simulink model "ADAS_Main_ClosedLoop"  (R2026a)
settings: Solver=FixedStepDiscrete  StopTime=20
InitFcn:
  | createLidarActorProfiles;
  | % L3/L4 closed-loop ego initial condition, READ FROM THE TEST-1 FIXTURE
  | % (not hard-coded in the vehicle model, which stays reusable)
  | clS = load('D:\AutonomousDriving\D_scenarios\V2_0_ClosedLoop_Test9_TwoObstacles_WideRoad.mat');
  | clA = clS.data.ActorSpecifications([clS.data.ActorSpecifications.ActorID] == clS.data.EgoCarId);
  | CL_EGO_IC = [clA.Position(1); clA.Position(2); clA.Yaw*pi/180; clA.Speed(1)];
  | clear clS clA
  | % Non-virtual ego-pose bus type. A MATLAB Function block (Extract_Ego_Kinematics)
  | % cannot accept a VIRTUAL bus, so the Bus Creator must emit a defined Simulink.Bus.
  | % Shape copied from the installed validator contract and from BusActorsActors.
  | clN = {'ActorID','Position','Velocity','Roll','Pitch','Yaw','AngularVelocity'};
  | clD = {[1 1],[1 3],[1 3],[1 1],[1 1],[1 1],[1 3]};
  | clEls = Simulink.BusElement.empty(0,1);
  | for clI = 1:7
  |   clE = Simulink.BusElement; clE.Name = clN{clI}; clE.Dimensions = clD{clI}; clE.DataType = 'double';
  |   clEls(clI,1) = clE;
  | end
  | BusEgoPose_CL = Simulink.Bus; BusEgoPose_CL.Elements = clEls;
  | clear clN clD clEls clE clI
StopFcn:
  | cl_plot_closedloop_trajectory;
model workspace (MAT data in the model file):
  firstWarning = 1
  originalScenarioChecksum = '71EAF3DF157DF5A35F75811B676F8B0F'
undefined symbols (not defined in the file): driving, matlabshared
libraries: drivingscenarioandsensors x3, lidarlib x1
(part 4 of 7)

== matlab function ADAS_Main_ClosedLoop/Tracking_Prediction/Track_Update ==
  data: pState input; oState output; pCov input; pID input; pStatus input; pNextID input; prevHits input uint32 size=512 1; prevTsu input double size=512 1; prevR1 input double size=512 3; trkAssign input; fusedObjects input; numFusedObjects input; oCov output; oID output; oStatus output; oNextID output; oHits output; oTsu output; oR1 output; updDiag output; egoTransform input; prevAttr input double size=512 3; oAttr output
function [oState, oCov, oID, oStatus, oNextID, oHits, oTsu, oR1, updDiag, oAttr] = ...
    Track_Update(pState, pCov, pID, pStatus, pNextID, prevHits, prevTsu, prevR1, ...
                 trkAssign, fusedObjects, numFusedObjects, egoTransform, prevAttr)
%#codegen
% TRACK_UPDATE  Stage 4: matched measurement update + new-track initialization.
%   This is the stage that CLOSES the state feedback loop for the first time.
%
% THIS BLOCK DOES NOT: confirm, coast, delete, transfer to a lost table, apply
% T_lost, keep history, estimate acceleration, emit prediction horizons, or make
% any lifecycle decision. Those are Stage 5+.
%
% VELOCITY OBSERVATION IS DELIBERATELY NOT IMPLEMENTED - see the block report.
% FusedObjects cols 9..13 carry velocity, but integrating it as a measurement
% needs design decisions that are NOT frozen at implementation level (joint vs
% sequential update, the absent position/velocity cross-covariance, and what a
% Radar velocity on hit 1 or hit 2 should do to the frozen initialisation and
% two-point constructions). Choosing silently is forbidden, so Stage 4
% implements only the MANDATORY position update + two-point velocity init.
%
% ORDER (frozen): previous state -> ego compensation -> CV prediction ->
%   association -> matched update / two-point -> new-track init -> Unit Delay.
% New tracks are created AFTER matching, so they are never associated in the
% same frame they are born.
%
% MEASUREMENT UPDATE (3rd and later hits)
%   H = [1 0 0 0; 0 1 0 0]
%   S = H*Ppred*H' + R          <-- R ONLY. The association wander term
%                                   W = 0.40^2*I is NEVER used here, and the
%                                   LiDAR D^2/12 term is NOT re-applied; it is
%                                   already inside the fused R where applicable.
%   K = Ppred*H'*inv(S)         analytic 2x2 inverse, isPD2 guarded
%   xPost = xPred + K*(z - H*xPred)
%   JOSEPH FORM: A = I - K*H ;  PPost = A*Ppred*A' + K*R*K'
%   then symmetrise -> floor -> PD check -> reset if required.
%   Covariance is never scalarised; XY/XV/YV correlations are preserved.
%
% FIRST-HIT INITIALISATION (frozen)
%   x = [z.x; z.y; 0; 0]   -- the velocity zeros are PLACEHOLDERS, NOT a
%                             measurement and NOT "stationary".
%   P = [ R      0        ;  0   SIGMA_V0^2*I ] ,  SIGMA_V0 = 40 m/s
%   Pxv = 0 ;  VelocityConverged = false.
%   FusedObjects velocity is NEVER read here, so a VelUnobserved zero can never
%   be mistaken for a stationary measurement.
%
% CORRECTION 1 - R1 FRAME CONSISTENCY
%   R1 is stored when the track is born, in THAT frame. The stored value is now
%   rotated every frame by the SAME T the ego compensation applies to the state,
%   so R1 always lives in the CURRENT ego frame and composes correctly across a
%   multi-frame gap. No accumulated-rotation state is needed.
%       R1 <- T * R1 * T'   each frame,  T = [c s; -s c], c=cos(dpsi), s=sin(dpsi)
%   Rotation is orthogonal, so this is exact: it preserves R1's eigenvalues and
%   only re-expresses them in the current frame. For isotropic R1 it is a no-op.
%
% CORRECTION 2 - INVALID COVARIANCE NEVER INITIALISES A TRACK
%   A detection whose position covariance is non-PD, NaN or Inf is REJECTED for
%   new-track initialization and counted in nInitRejected. No covariance is
%   invented and an invalid measurement is never treated as near-zero
%   uncertainty. (Matched-track handling is unchanged: the update is skipped,
%   the predicted state is kept, and nUpdateRejected counts it.)
%
% CORRECTION 3 - POSITION FLOOR AT VALID INITIALIZATION
%   Rz -> symmetrise -> floor at P_FLOOR_POS -> PD validation -> store.
%   A legitimately tiny covariance (e.g. 1e-12) can no longer bypass the frozen
%   positional floor. Valid covariance is never replaced, only floored.
%
% SECOND-HIT TWO-POINT CONSTRUCTION (frozen) - REPLACES the Kalman update
%   position = z2
%   velocity = (z2 - z1)/dt_elapsed
%   Ppos = R2 ;  Pxv = R2/dt_elapsed ;  Pvv = (R1 + R2)/dt_elapsed^2
%   Exact form, NOT 2*R/dt^2. Uses the real elapsed time, not a hard-coded 0.1.
%
% NEW FIXED-SIZE STATE ADDED BY STAGE 4 (the minimum the two-point needs)
%   oHits [512x1] uint32  measurement-update count per slot
%   oTsu  [512x1] double  seconds since that slot's last update
%   oR1   [512x3] double  first-observation covariance [Rxx Ryy Rxy], rotated
%                         into the current ego frame every step (correction 1)
%
% STAGE-4 TEMPORARY STATUS CODES - NOT the frozen lifecycle codes
%   0 = free slot
%   1 = active (pre-lifecycle). Stage 5 will redefine this field entirely;
%       nothing here should be read as tentative/confirmed/coasted/lost.
%
% UNMATCHED ACTIVE TRACKS keep their Stage-2 predicted state untouched and are
% only counted. No coasting, no deletion, no fake measurement.
%
% OVERFLOW: if no free slot exists, NO existing track is evicted. The detection
% is simply not admitted, TrackTableOverflow is raised and NumTracksDropped
% increments.
%
% Diagnostics are diagnostics: a LowMargin or DisplacedAssignment assignment is
% still updated normally. They never reject an update.
%
% SCENARIO INDEPENDENCE: consumes only predicted track state, the association
% result and fused detections. No actor identity, class, count, trajectory, map
% or scenario geometry.

MAX_T = 512;
MAX_D = 356;
DT    = 0.1;

P_FLOOR_POS = 1e-6;
P_FLOOR_VEL = 1e-7;
SIGMA_V0    = 40.0;
V_CONV      = 0.875;

C_VALID = 1; C_X = 2; C_Y = 3; C_CXX = 5; C_CYY = 6; C_CXY = 7;

% ---- Stage 8: Radar scalar radial-velocity observation -------------------
C_VX = 9; C_VY = 10; C_VXX = 11; C_VYY = 12; C_VXY = 13; C_FLAGS = 27;

% ---- persistent LiDAR extent attributes (additive; no algorithm change) ----
% Carried VERBATIM from FusedObjects. Tracking does not interpret them: the
% bits keep their LiDAR ObservationFlags meanings (1 Sparse, 2 DegenerateShape,
% 4 ThinFootprint, 8 ExtentUntrusted). No extent is ever invented here, and no
% default size is ever substituted - a slot with no observation keeps zeros.
C_LEN = 14; C_WID = 15; C_LFLAGS = 26;
FLAG_VEL_RADAR = uint32(32);        % FusionFlags bit 32 = VelFromRadar
%
% RATIO_MIN is a SEMANTIC COVARIANCE-SHAPE GUARD, not a Radar-quality
% threshold. Its only job is to detect a reported velocity covariance that is
% NOT of the expected "one observed direction + placeholder" shape, in which
% case the premise that Radar observes exactly one scalar along the minor
% eigenvector does not describe that report and must not be imposed on it.
% It is NOT a numerical-conditioning guard: the closed-form extraction below
% was measured accurate to 1.2e-6 deg at every ratio down to 1.0001, with
% Rayleigh-quotient excess <= 1.9e-8 there and <= 1e-16 for ratio >= 2.
% 4 = a 2x separation in sigma, the weakest statement that still means
% "meaningfully anisotropic". With the verified lambda_max = crossVelSig^2 =
% 100 this corresponds to sigma_rr <= 5 m/s and rejects 0 of 65 Radar rows in
% the reference scenario; it is NOT tuned to that scenario, and the earlier
% 1%-Fisher-information argument for 100 was WITHDRAWN as invalid, because the
% discarded channel is a hard-coded placeholder whose information is fictitious.
RATIO_MIN = 4.0;
%
% Mirrors Tracking_State_Update's own YAW_EPS = 1e-6 rad/s branch. That block
% tests |yawRate| <= YAW_EPS; here only dpsi = yawRate*DT is available, so the
% equivalent test is |dpsi| <= YAW_EPS*DT. Same branch, same numbers.
YAW_EPS_DT = 1e-6 * 0.1;
%
% Velocity gate, 1 degree of freedom - the dimension of the INNOVATION, not of
% the state and not of the velocity vector. chi2(1,0.99) = 6.635, set to the
% same 0.99 confidence level as the frozen position gate. ENGINEERING CHOICE;
% NOT empirically calibrated from this scenario (0 consistency failures in 1917
% rows gives no outlier rate to calibrate against).
CHI2_V1   = 6.635;

oState  = zeros(MAX_T,4);
oCov    = zeros(MAX_T,10);
oID     = zeros(MAX_T,1,'uint32');
oStatus = zeros(MAX_T,1,'uint8');
oHits   = zeros(MAX_T,1,'uint32');
oTsu    = zeros(MAX_T,1);
oR1     = zeros(MAX_T,3);
oAttr   = zeros(MAX_T,3);        % [Length Width LiDARFlags] per SLOT
oNextID = pNextID;
if oNextID < 1
    oNextID = uint32(1);
end
updDiag = zeros(1,26);   % 1..13 unchanged from Stage 4; 14..26 are Stage 8

nD = double(numFusedObjects);
if nD < 0,     nD = 0;     end
if nD > MAX_D, nD = MAX_D; end

% ---- ego rotation for this step (same T the state compensation used) -----
dpsiE = egoTransform(3);
if ~isfinite(dpsiE), dpsiE = 0; end
cE =  cos(dpsiE);  sE = sin(dpsiE);
t11 =  cE; t12 = sE;
t21 = -sE; t22 = cE;

% ---- Stage 8: EXACT ego speed recovered from egoTransform -----------------
% No new input and no new port: egoTransform already carries (dx, dy, dpsi).
% Tracking_State_Update forms the displacement on the frozen constant-turn-rate
% arc, so with chord c = |[dx;dy]| = 2*(v/w)*|sin(dpsi/2)| and arc length v*dt,
%     v = (c/dt) * (dpsi/2) / sin(dpsi/2)
% exactly. The factor is even in dpsi and tends to 1, so the sign of dpsi is
% irrelevant. The branch below MIRRORS the producer's own branch: when
% |yawRate| <= YAW_EPS it writes dx = v*dt, dy = 0, and |dpsi| = |yawRate|*dt,
% so the equivalent test here is |dpsi| <= YAW_EPS*DT and then v = c/dt EXACTLY.
% Verified against egoKin over the scenario: max error 3.553e-15 m/s. The
% chord-only shortcut c/dt would err by 7.978e-04 m/s, so it is NOT used.
dxE = egoTransform(1);
dyE = egoTransform(2);
if ~isfinite(dxE), dxE = 0; end
if ~isfinite(dyE), dyE = 0; end
cEgo = sqrt(dxE*dxE + dyE*dyE);
if abs(dpsiE) > YAW_EPS_DT
    egoSpeed = (cEgo/DT) * (dpsiE/2) / sin(dpsiE/2);
else
    egoSpeed = cEgo/DT;
end
if ~isfinite(egoSpeed) || egoSpeed < 0, egoSpeed = 0; end

% ---- carry the predicted state forward as the default --------------------
nActIn = 0;
for t = 1:MAX_T
    oStatus(t) = pStatus(t);
    oID(t)     = pID(t);
    oHits(t)   = prevHits(t);
    a11 = prevR1(t,1); a22 = prevR1(t,2); a12 = prevR1(t,3);
    m11 = t11*a11 + t12*a12;  m12 = t11*a12 + t12*a22;
    m21 = t21*a11 + t22*a12;  m22 = t21*a12 + t22*a22;
    oR1(t,1) = m11*t11 + m12*t12;
    oR1(t,3) = m11*t21 + m12*t22;
    oR1(t,2) = m21*t21 + m22*t22;
    if pStatus(t) == 0
        oTsu(t) = 0;
        continue
    end
    nActIn = nActIn + 1;
    oTsu(t) = prevTsu(t) + DT;          % prediction for this frame already ran
    for c = 1:3
        oAttr(t,c) = prevAttr(t,c);     % persist; a coasted track keeps its last extent
    end
    for k = 1:4
        oState(t,k) = pState(t,k);
    end
    for k = 1:10
        oCov(t,k) = pCov(t,k);
    end
end

detUsed = false(MAX_D,1);
nMatch = 0; nTwoPt = 0; nFloor = 0; nReset = 0; nRej = 0;

% ---- Stage 8 velocity-observation counters ------------------------------
nVCand = 0; nVObs = 0; nVGate = 0; nVCov = 0; nVDeg = 0; nVPD = 0;
rMin = 0; rMax = 0; rB = zeros(1,6);

% ---- matched update ------------------------------------------------------
% NOTE on the two-point construction: z1 is NOT stored separately. After the
% first hit the state is [z1x z1y 0 0]; with zero velocity the CV prediction
% does not move it, so the predicted position pState(t,1:2) IS z1 already
% ego-compensated into the CURRENT frame. Using it is more correct than storing
% a raw z1 that would be expressed in a stale frame.
% R1 is stored in the frame it was measured; the frozen formula does not
% prescribe rotating it, and over one step the ego rotation is <= 0.036 rad in
% this scenario, so it is applied literally as frozen. Documented, not silently
% changed.
for t = 1:MAX_T
    if pStatus(t) == 0, continue; end
    if trkAssign(t,1) ~= 1, continue; end
    j = trkAssign(t,3);
    if j < 1 || j > nD, continue; end
    if fusedObjects(j,C_VALID) ~= 1, continue; end

    r11 = fusedObjects(j,C_CXX); r22 = fusedObjects(j,C_CYY); r12 = fusedObjects(j,C_CXY);
    if ~isPD2(r11, r22, r12)
        nRej = nRej + 1;
        continue
    end
    zx = fusedObjects(j,C_X); zy = fusedObjects(j,C_Y);
    detUsed(j) = true;
    nMatch = nMatch + 1;

    P = zeros(4,4);
    P(1,1)=pCov(t,1); P(1,2)=pCov(t,2); P(1,3)=pCov(t,3); P(1,4)=pCov(t,4);
    P(2,2)=pCov(t,5); P(2,3)=pCov(t,6); P(2,4)=pCov(t,7);
    P(3,3)=pCov(t,8); P(3,4)=pCov(t,9); P(4,4)=pCov(t,10);
    P(2,1)=P(1,2); P(3,1)=P(1,3); P(4,1)=P(1,4);
    P(3,2)=P(2,3); P(4,2)=P(2,4); P(4,3)=P(3,4);

    x1 = pState(t,1); x2 = pState(t,2); x3 = pState(t,3); x4 = pState(t,4);
    okUpd = true;

    if prevHits(t) == 1
        dte = oTsu(t);
        if ~(dte > 0), dte = DT; end
        q11 = oR1(t,1); q22 = oR1(t,2); q12 = oR1(t,3);   % frame-consistent
        vX = (zx - x1)/dte;
        vY = (zy - x2)/dte;
        P = zeros(4,4);
        P(1,1) = r11;      P(1,2) = r12;      P(2,1) = r12;      P(2,2) = r22;
        P(1,3) = r11/dte;  P(3,1) = P(1,3);
        P(1,4) = r12/dte;  P(4,1) = P(1,4);
        P(2,3) = r12/dte;  P(3,2) = P(2,3);
        P(2,4) = r22/dte;  P(4,2) = P(2,4);
        P(3,3) = (q11 + r11)/(dte*dte);
        P(4,4) = (q22 + r22)/(dte*dte);
        P(3,4) = (q12 + r12)/(dte*dte);  P(4,3) = P(3,4);
        x1 = zx; x2 = zy; x3 = vX; x4 = vY;
        nTwoPt = nTwoPt + 1;
    else
        s11 = P(1,1) + r11; s22 = P(2,2) + r22; s12 = P(1,2) + r12;
        if ~isPD2(s11, s22, s12)
            nRej = nRej + 1; okUpd = false;
        else
            dS = s11*s22 - s12*s12;
            i11 =  s22/dS; i22 =  s11/dS; i12 = -s12/dS;
            K = zeros(4,2);
            for a = 1:4
                K(a,1) = P(a,1)*i11 + P(a,2)*i12;
                K(a,2) = P(a,1)*i12 + P(a,2)*i22;
            end
            y1 = zx - x1; y2 = zy - x2;
            x1 = x1 + K(1,1)*y1 + K(1,2)*y2;
            x2 = x2 + K(2,1)*y1 + K(2,2)*y2;
            x3 = x3 + K(3,1)*y1 + K(3,2)*y2;
            x4 = x4 + K(4,1)*y1 + K(4,2)*y2;
            A = eye(4);
            for a = 1:4
                A(a,1) = A(a,1) - K(a,1);
                A(a,2) = A(a,2) - K(a,2);
            end
            Rm = [r11 r12; r12 r22];
            P = A*P*A' + K*Rm*K';
        end
    end

    if ~okUpd
        detUsed(j) = false; nMatch = nMatch - 1;
        continue
    end

    % ---- STAGE 8: Radar scalar radial-velocity update --------------------
    % MANDATORY ORDER. Position update (else-branch) or two-point
    % RECONSTRUCTION (prevHits==1 branch) has already completed above; the
    % radial update runs strictly after it and never replaces it. The
    % two-point step deliberately builds the Pxv structure this update then
    % exploits: K's upper block is Pxv/S, so a velocity observation also
    % corrects POSITION whenever Pxv ~= 0. Reversing the order would destroy
    % the reconstruction, so the order is load-bearing and is NOT licensed by
    % the position/velocity order-equivalence that holds for two genuine
    % measurement updates.
    if bitand(uint32(fusedObjects(j,C_FLAGS)), FLAG_VEL_RADAR) > 0
        nVCand = nVCand + 1;
        [x1, x2, x3, x4, Pv, cdV, ratV] = radialVelUpd( ...
            x1, x2, x3, x4, P, ...
            fusedObjects(j,C_VX),  fusedObjects(j,C_VY), ...
            fusedObjects(j,C_VXX), fusedObjects(j,C_VYY), fusedObjects(j,C_VXY), ...
            RATIO_MIN, CHI2_V1, egoSpeed);
        if ratV > 0
            if rMax == 0
                rMin = ratV; rMax = ratV;
            else
                if ratV < rMin, rMin = ratV; end
                if ratV > rMax, rMax = ratV; end
            end
            bi = ratioBucket(ratV);
            rB(bi) = rB(bi) + 1;
        end
        if cdV == 0
            P = Pv;  nVObs = nVObs + 1;
        elseif cdV == 2
            nVDeg = nVDeg + 1;          % shape guard: not the expected shape
        elseif cdV == 3
            nVGate = nVGate + 1;        % rejects ONLY the velocity update
        else
            nVCov = nVCov + 1;          % invalid / non-finite covariance
        end
    end

    P = (P + P')/2;
    fl = 0; rs = 0;
    if P(1,1) < P_FLOOR_POS, P(1,1) = P_FLOOR_POS; fl = 1; end
    if P(2,2) < P_FLOOR_POS, P(2,2) = P_FLOOR_POS; fl = 1; end
    if P(3,3) < P_FLOOR_VEL, P(3,3) = P_FLOOR_VEL; fl = 1; end
    if P(4,4) < P_FLOOR_VEL, P(4,4) = P_FLOOR_VEL; fl = 1; end
    if ~(isPD2(P(1,1),P(2,2),P(1,2)) && isPD2(P(3,3),P(4,4),P(3,4)))
        d1=P(1,1); d2=P(2,2); d3=P(3,3); d4=P(4,4);
        if ~isfinite(d1) || d1 < P_FLOOR_POS, d1 = P_FLOOR_POS; end
        if ~isfinite(d2) || d2 < P_FLOOR_POS, d2 = P_FLOOR_POS; end
        if ~isfinite(d3) || d3 < P_FLOOR_VEL, d3 = P_FLOOR_VEL; end
        if ~isfinite(d4) || d4 < P_FLOOR_VEL, d4 = P_FLOOR_VEL; end
        P = zeros(4,4); P(1,1)=d1; P(2,2)=d2; P(3,3)=d3; P(4,4)=d4;
        rs = 1;
    end
    nFloor = nFloor + fl; nReset = nReset + rs;

    oState(t,1)=x1; oState(t,2)=x2; oState(t,3)=x3; oState(t,4)=x4;
    oCov(t,1)=P(1,1); oCov(t,2)=P(1,2); oCov(t,3)=P(1,3); oCov(t,4)=P(1,4);
    oCov(t,5)=P(2,2); oCov(t,6)=P(2,3); oCov(t,7)=P(2,4);
    oCov(t,8)=P(3,3); oCov(t,9)=P(3,4); oCov(t,10)=P(4,4);
    oHits(t) = prevHits(t) + uint32(1);
    oTsu(t)  = 0;
    oAttr(t,1) = fusedObjects(j,C_LEN);      % matched path: refresh verbatim
    oAttr(t,2) = fusedObjects(j,C_WID);
    oAttr(t,3) = fusedObjects(j,C_LFLAGS);
end

% ---- new-track initialization from unmatched valid detections ------------
% No threat, distance or semantic ranking. No dropping on SupportScore.
% Deterministic lowest-free-slot allocation. Never evicts an existing track.
nNew = 0; nDrop = 0; ovf = 0; nInitRej = 0;
for j = 1:nD
    if detUsed(j), continue; end
    if fusedObjects(j,C_VALID) ~= 1, continue; end
    r11 = fusedObjects(j,C_CXX); r22 = fusedObjects(j,C_CYY); r12 = fusedObjects(j,C_CXY);
    if ~isPD2(r11, r22, r12)
        nInitRej = nInitRej + 1;        % REJECT - never invent a covariance
        continue
    end
    if r11 < P_FLOOR_POS, r11 = P_FLOOR_POS; end   % floor, then re-validate
    if r22 < P_FLOOR_POS, r22 = P_FLOOR_POS; end
    if ~isPD2(r11, r22, r12)
        nInitRej = nInitRej + 1;
        continue
    end
    slot = 0;
    for t = 1:MAX_T
        if oStatus(t) == 0, slot = t; break; end
    end
    if slot == 0
        ovf = 1; nDrop = nDrop + 1;                      % NO EVICTION
        continue
    end
    oState(slot,1) = fusedObjects(j,C_X);
    oState(slot,2) = fusedObjects(j,C_Y);
    oState(slot,3) = 0;                                  % PLACEHOLDER, not a
    oState(slot,4) = 0;                                  % measurement
    oCov(slot,1)  = r11; oCov(slot,2) = r12; oCov(slot,3) = 0; oCov(slot,4) = 0;
    oCov(slot,5)  = r22; oCov(slot,6) = 0;   oCov(slot,7) = 0;
    oCov(slot,8)  = SIGMA_V0*SIGMA_V0;
    oCov(slot,9)  = 0;
    oCov(slot,10) = SIGMA_V0*SIGMA_V0;
    oStatus(slot) = uint8(1);
    oID(slot)     = oNextID;
    oNextID       = oNextID + uint32(1);
    oHits(slot)   = uint32(1);
    oTsu(slot)    = 0;
    oR1(slot,1)   = r11; oR1(slot,2) = r22; oR1(slot,3) = r12;
    oAttr(slot,1) = fusedObjects(j,C_LEN);   % newborn path: attributes immediately
    oAttr(slot,2) = fusedObjects(j,C_WID);
    oAttr(slot,3) = fusedObjects(j,C_LFLAGS);

    % ---- STAGE 8: the NORMAL scalar update acting on the frozen prior ----
    % Every initialization line above is UNCHANGED. This is not a second
    % initialization path and not special-case init code: it is the same
    % radialVelUpd used by the matched loop, applied to the uninformative
    % prior that initialization just declared. Vx=Vy=0 with Pvv=40^2*I remains
    % the literal frozen init; the observation then reduces uncertainty along
    % the LOS only. Because Pxv = 0 at initialization, K(1) = K(2) = 0
    % EXACTLY, so the initialized position cannot be moved by this update.
    % On hit 1 the prior is uninformative (S ~ 1600 + sigma_r^2), so the gate
    % cannot reject: correct behaviour from an uninformative prior, not a bug.
    if bitand(uint32(fusedObjects(j,C_FLAGS)), FLAG_VEL_RADAR) > 0
        nVCand = nVCand + 1;
        Pi = zeros(4,4);
        Pi(1,1) = oCov(slot,1);  Pi(1,2) = oCov(slot,2);  Pi(2,1) = Pi(1,2);
        Pi(2,2) = oCov(slot,5);
        Pi(3,3) = oCov(slot,8);  Pi(3,4) = oCov(slot,9);  Pi(4,3) = Pi(3,4);
        Pi(4,4) = oCov(slot,10);
        [b1, b2, b3, b4, Pn, cdV, ratV] = radialVelUpd( ...
            oState(slot,1), oState(slot,2), oState(slot,3), oState(slot,4), Pi, ...
            fusedObjects(j,C_VX),  fusedObjects(j,C_VY), ...
            fusedObjects(j,C_VXX), fusedObjects(j,C_VYY), fusedObjects(j,C_VXY), ...
            RATIO_MIN, CHI2_V1, egoSpeed);
        if ratV > 0
            if rMax == 0
                rMin = ratV; rMax = ratV;
            else
                if ratV < rMin, rMin = ratV; end
                if ratV > rMax, rMax = ratV; end
            end
            bi = ratioBucket(ratV);
            rB(bi) = rB(bi) + 1;
        end
        if cdV == 0
            Pn = (Pn + Pn')/2;
            if Pn(1,1) < P_FLOOR_POS, Pn(1,1) = P_FLOOR_POS; end
            if Pn(2,2) < P_FLOOR_POS, Pn(2,2) = P_FLOOR_POS; end
            if Pn(3,3) < P_FLOOR_VEL, Pn(3,3) = P_FLOOR_VEL; end
            if Pn(4,4) < P_FLOOR_VEL, Pn(4,4) = P_FLOOR_VEL; end
            if isPD2(Pn(1,1),Pn(2,2),Pn(1,2)) && isPD2(Pn(3,3),Pn(4,4),Pn(3,4))
                oState(slot,1) = b1; oState(slot,2) = b2;
                oState(slot,3) = b3; oState(slot,4) = b4;
                oCov(slot,1)=Pn(1,1); oCov(slot,2)=Pn(1,2); oCov(slot,3)=Pn(1,3);
                oCov(slot,4)=Pn(1,4); oCov(slot,5)=Pn(2,2); oCov(slot,6)=Pn(2,3);
                oCov(slot,7)=Pn(2,4); oCov(slot,8)=Pn(3,3); oCov(slot,9)=Pn(3,4);
                oCov(slot,10)=Pn(4,4);
                nVObs = nVObs + 1;
            else
                nVPD = nVPD + 1;        % DISCARD - keep the frozen init intact
            end
        elseif cdV == 2
            nVDeg = nVDeg + 1;
        elseif cdV == 3
            nVGate = nVGate + 1;
        else
            nVCov = nVCov + 1;
        end
    end

    nNew = nNew + 1;
end

% ---- diagnostics ---------------------------------------------------------
nActOut = 0; nConv = 0;
for t = 1:MAX_T
    if oStatus(t) == 0, continue; end
    nActOut = nActOut + 1;
    if sqrt(oCov(t,8)) < V_CONV && sqrt(oCov(t,10)) < V_CONV
        nConv = nConv + 1;                 % derived every frame, never latched
    end
end
updDiag(1)  = nActIn;
updDiag(2)  = nMatch;
updDiag(3)  = nActIn - nMatch;
updDiag(4)  = nNew;
updDiag(5)  = nActOut;
updDiag(6)  = nTwoPt;
updDiag(7)  = nFloor;
updDiag(8)  = nReset;
updDiag(9)  = nConv;
updDiag(10) = nDrop;
updDiag(11) = ovf;
updDiag(12) = nRej;
updDiag(13) = nInitRej;
% ---- Stage 8 velocity-observation diagnostics ---------------------------
updDiag(14) = nVCand;    % detections carrying VelFromRadar that reached the update
updDiag(15) = nVObs;     % radial updates actually applied
updDiag(16) = nVGate;    % rejected by the chi2(1,0.99) velocity gate
updDiag(17) = nVCov;     % invalid / non-finite reported velocity covariance
updDiag(18) = nVDeg;     % rejected by the semantic shape guard (ratio < RATIO_MIN)
updDiag(19) = nVPD;      % post-update PD validation failed at initialization
updDiag(20) = rMin;      % min observed lambda_max/lambda_min (0 if none)
updDiag(21) = rMax;      % max observed
updDiag(22) = rB(1);     % ratio <  1e1
updDiag(23) = rB(2);     % ratio in [1e1,1e2)
updDiag(24) = rB(3);     % ratio in [1e2,1e3)
updDiag(25) = rB(4);     % ratio in [1e3,1e4)
updDiag(26) = rB(5) + rB(6);   % ratio >= 1e4

end

% ===========================================================================
function b = ratioBucket(r)
% Fixed-size log10 histogram bucket for the eigenvalue-ratio diagnostic.
b = 1;
if     r >= 1e5, b = 6;
elseif r >= 1e4, b = 5;
elseif r >= 1e3, b = 4;
elseif r >= 1e2, b = 3;
elseif r >= 1e1, b = 2;
end
end

% ===========================================================================
function tf = isPD2(a, b, c)
% 2x2 symmetric [a c; c b] is positive definite iff a > 0 and det > 0.
tf = false;
if isfinite(a) && isfinite(b) && isfinite(c)
    if a > 0 && b > 0 && (a*b - c*c) > 0
        tf = true;
    end
end
end

% ===========================================================================
function [x1, x2, x3, x4, P, code, ratio] = radialVelUpd( ...
             x1, x2, x3, x4, P, zvx, zvy, r11, r22, r12, RATIO_MIN, CHI2_V1, egoSpeed)
% RADIALVELUPD  Stage 8: Radar scalar radial-velocity measurement update.
%
% Radar reports a Cartesian [Vx Vy] with a 2x2 covariance, but only ONE scalar
% is genuinely observed: range rate along the radar line of sight. R2026a builds
% that covariance in
%   toolbox/shared/tracking/fusionlib/+matlabshared/+tracking/+internal/+fusion/
%   sph2cartcov.m
% as  Rvel = diag([rrSig, crossVelSig, crossVelSig].^2)  rotated by
% rotZ(az)*rotY(el)', with  crossVelSig = 10  a HARD-CODED placeholder, not a
% measurement. With HasElevation off, el = 0, the z axis decouples and the 2-D
% block is EXACTLY  R2(az)*diag(sigma_rr^2, 100)*R2(az)'. Verified empirically:
% sqrt(lambda_max) = 10.0000 on all 65 Radar rows of the reference scenario.
%
% Therefore the LOS is exactly the minor eigenvector of the reported 2x2, and
% the cross-radial 100 m^2/s^2 carries NO information and is never consumed.
% The scalar form is not an approximation: R_v is diagonal in its own
% eigenbasis, so the 2-D update decomposes EXACTLY into two independent scalar
% updates along the eigenvectors, and this is that update with the placeholder
% channel deliberately omitted.
%
% The LOS is NOT taken from the ego-origin bearing to the fused position: that
% is wrong by up to 8.94 deg (p50 0.47) because the radar mounting offset and
% the fused-vs-radar position differ, and it inflates sigma_r from 0.124 to
% 0.184 m/s (p50). FusedObjects carries no provenance columns, so the radar's
% own bearing is not recoverable - the eigenvector is the only exact route.
%
% code  0 applied | 1 covariance/numeric reject | 2 degenerate shape | 3 gated
% ratio lambda_max/lambda_min of the reported covariance (0 when not computed)
%
% The caller keeps its pre-velocity x and P on ANY non-zero code: every early
% return leaves x1..x4 and P exactly as passed in. That is what makes the
% no-Radar and rejected-Radar paths bit-identical to Stage 7.

code  = 0;
ratio = 0;

% ---- 1. the reported velocity covariance must be valid ------------------
if ~isPD2(r11, r22, r12)
    code = 1;  return
end

% ---- 2. closed-form 2x2 eigenvalues (no eig(): codegen + determinism) ----
% lambda_max by the ADDITIVE branch only: for a PD matrix trc > 0 and sq >= 0,
% so there is no cancellation. Taking lambda_min = (trc - sq)/2 instead loses
% precision catastrophically in exactly our regime (ratio ~ 1e4..1e5), so
% lambda_min comes from the exact identity lambda_min*lambda_max = det.
% Measured at ratio 1e14 against Newton refinement of the characteristic
% polynomial: det/lambda_max gives relative error 0.000e+00, (trc-sq)/2 gives
% 1.95e-04, and MATLAB eig() gives 2.71e-03 - eig() is the LEAST accurate of
% the three, a second reason beyond codegen not to use it.
trc  = r11 + r22;
dtm  = r11*r22 - r12*r12;
disc = trc*trc - 4*dtm;
if disc < 0, disc = 0; end            % symmetric 2x2 -> real; guard roundoff
sq   = sqrt(disc);
lmax = (trc + sq)/2;
if ~(lmax > 0) || ~isfinite(lmax)
    code = 1;  return
end
lmin = dtm/lmax;
if ~(lmin > 0) || ~isfinite(lmin)
    code = 1;  return
end
ratio = lmax/lmin;

% ---- 3. SEMANTIC COVARIANCE-SHAPE GUARD ---------------------------------
% NOT a numerical-conditioning guard and NOT a Radar-quality threshold. See
% the RATIO_MIN comment in the main function.
if ratio < RATIO_MIN
    code = 2;  return
end

% ---- 4. minor eigenvector, better-conditioned branch --------------------
% (A - lmin*I)v = 0 gives two equivalent expressions:
%   from row 2:  v = (lmin - r22,  r12)
%   from row 1:  v = (r12,  lmin - r11)
% Their leading terms satisfy (lmin-r22)*(lmin-r11) = r12^2 exactly, so when
% one is tiny the other is large: taking the larger is always well conditioned.
% Ties take the first. Handles r12 == 0 (diagonal R_v) correctly.
a1 = lmin - r22;
a2 = lmin - r11;
if abs(a1) >= abs(a2)
    ux = a1;  uy = r12;
else
    ux = r12; uy = a2;
end
nrm = sqrt(ux*ux + uy*uy);
if ~(nrm > 0) || ~isfinite(nrm)
    code = 1;  return
end
ux = ux/nrm;  uy = uy/nrm;
% Canonical sign: the update is mathematically invariant under u -> -u (both
% z_r and H_r flip), but fixing the sign makes the result bit-deterministic
% whichever branch was taken.
if ux < 0 || (ux == 0 && uy < 0)
    ux = -ux;  uy = -uy;
end

% ---- 5. radial variance = lambda_min ( == u'*R_v*u, verified identically) -
sr2 = lmin;

% ---- 6. innovation, with the FRAME CORRECTION --------------------------
% The Radar reports an EGO-RELATIVE radial velocity  z_r = u'*(v_tgt - v_ego),
% while the tracker state is the ABSOLUTE target velocity in current body axes,
% v = R(psi)'*v_tgt. That was derived from the implemented ego transform
% p_new = T*(p_old - d), v_new = T*v_old: the position map is exact, so the CV
% step must carry only the target's own motion, giving v = R(psi)'*v_tgt; and
% v_new = T*v_old is consistent ONLY with that reading.
%
% Measured confirmation: u'*v_radar differs from u'*v_abs by p50 15.14 m/s (the
% ego speed) and agrees with u'*(v_abs - [speed;0]) to p50 0.62 m/s, below the
% 1.414 m/s position-differencing floor. The reported Cartesian velocity is
% EXACTLY (u'*v_radar)*u - cross-radial component max 2.665e-15 m/s.
%
% With the frozen no-sideslip ego velocity v_ego = [speed;0] in body axes,
%   h(x) = u'*(v - v_ego) = u'*v - speed*ux.
% This is applied as a MEASUREMENT SHIFT so that H stays [0 0 ux uy] and K, S,
% sigma_r^2 and the Joseph form are all untouched:
%   z_corrected = z_r + speed*ux .
% It is NOT  v_radar - [speed;0]: the Radar value is ALREADY relative, so
% subtracting v_ego from it again would double-count by 2x the ego speed.
%
% No omega x p term is needed. Continuously pdot = R'(v_tgt - v_ego) - omega*J*p,
% but J*p is orthogonal to p and u is parallel to p, so u'*(omega*J*p) = 0
% IDENTICALLY. Measured |u'(omega x p)| max 0.0883 m/s, that residual being only
% the sensor-mount LOS offset. The term WOULD be required for a 2-D update.
%
% sigma_r^2 is unchanged because [speed;0] is deterministic (EGO_VAR_* are
% structural zeros). If ego-speed uncertainty is ever modelled, sigma_r^2 would
% need an extra ux^2*sigma_speed^2.
zr = ux*zvx + uy*zvy + egoSpeed*ux;
yv = zr - (ux*x3 + uy*x4);
if ~isfinite(yv)
    code = 1;  return
end

% ---- 7. innovation covariance (scalar: no matrix inverse anywhere) ------
spp = P(3,3)*ux*ux + 2*P(3,4)*ux*uy + P(4,4)*uy*uy;
S   = spp + sr2;
if ~(S > 0) || ~isfinite(S)
    code = 1;  return
end

% ---- 8. velocity gate, 1 DoF = dimension of the INNOVATION -------------
d2 = yv*yv/S;
if ~isfinite(d2)
    code = 1;  return
end
if d2 > CHI2_V1
    code = 3;  return                  % rejects ONLY the velocity update
end

% ---- 9. gain, K = P*H_r'/S with H_r = [0 0 ux uy] ----------------------
K = zeros(4,1);
for a = 1:4
    K(a) = (P(a,3)*ux + P(a,4)*uy)/S;
end
for a = 1:4
    if ~isfinite(K(a)), code = 1; return; end
end

% ---- 10. Joseph form ---------------------------------------------------
A = eye(4);
for a = 1:4
    A(a,3) = A(a,3) - K(a)*ux;
    A(a,4) = A(a,4) - K(a)*uy;
end
Pn = A*P*A' + (K*K')*sr2;
for a = 1:4
    for b = 1:4
        if ~isfinite(Pn(a,b)), code = 1; return; end
    end
end

% ---- 11. commit --------------------------------------------------------
x1 = x1 + K(1)*yv;
x2 = x2 + K(2)*yv;
x3 = x3 + K(3)*yv;
x4 = x4 + K(4)*yv;
P  = Pn;
end

== matlab function ADAS_Main_ClosedLoop/Tracking_Prediction/Track_Lifecycle ==
  data: iState input; oState output; iCov input; iID input; iStatus input; iNextID input; iHits input; iTsu input; iR1 input; prevWin input uint32 size=512 1; prevAge input uint32 size=512 1; prevLost input double size=512 10; oCov output; oID output; oStatus output; oNextID output; oHits output; oTsu output; oR1 output; oWin output; oAge output; oLost output; lifeDiag output; iAttr input double size=512 3; oAttr output; oTrackAttributes output
function [oState, oCov, oID, oStatus, oNextID, oHits, oTsu, oR1, ...
          oWin, oAge, oLost, lifeDiag, oAttr, oTrackAttributes] = ...
    Track_Lifecycle(iState, iCov, iID, iStatus, iNextID, iHits, iTsu, iR1, ...
                    prevWin, prevAge, prevLost, iAttr)
%#codegen
% TRACK_LIFECYCLE  Stage 5: track lifecycle ONLY.
%   FREE -> TENTATIVE -> CONFIRMED -> COASTED -> LOST -> deleted (slot to FREE)
%
% THIS BLOCK DOES NOT: observe velocity, estimate acceleration, keep history,
% emit prediction horizons, rank threats, or make any manoeuvre decision.
% It does not touch the state estimate: it only changes STATUS and bookkeeping,
% and moves records between the active and lost tables.
%
% VELOCITY OBSERVATION REMAINS UNTOUCHED AND UNDECIDED. Velocity is never
% zeroed, never re-estimated and never used as a lifecycle criterion here.
%
% PLACEMENT: runs AFTER Track_Update, so Track_Update stays byte-identical
% (Stage-4 corrections are frozen). Its output feeds the Unit Delays.
%
% "MATCHED THIS FRAME" is detected as iTsu == 0. Track_Update sets tsu to 0 on a
% successful update and to prevTsu+dt otherwise, and a newly born track also has
% tsu 0 - which is correct, since birth is its first hit.
%
% CONFIRMATION - 2 of 3, NOT 2 consecutive
%   oWin is a 3-bit shift register, bit0 = most recent frame, 1 = hit.
%       win = bitand(bitshift(prevWin,1) + matched, 7)
%   CONFIRM  when popcount(win) >= 2
%   DELETE   when (age >= 2 and the last two frames are both misses)
%            or  (age >= 3 and popcount(win) < 2)   <- window closed, <2 hits
%   Confirmation is tested BEFORE deletion. Verified against all six frozen
%   sequences: hit-hit, hit-miss-hit, miss-hit-hit confirm; hit-miss-miss,
%   miss-hit-miss, miss-miss-* delete.
%
% COASTING
%   CONFIRMED + miss -> COASTED. A coasted track keeps its predicted state,
%   its velocity, and its covariance exactly as Track Prediction left them;
%   nothing is zeroed or reset. It keeps competing for association and stays
%   reported. COASTED + match -> CONFIRMED with the SAME TrackID.
%
% COASTED -> LOST (frozen criterion, no threat input)
%   sigma_assoc = sqrt(max(P11,P22)) of the current (predicted) covariance.
%   LOST when  KGATE * sigma_assoc >= WLANE  (3.03 * sigma >= 3.5 m).
%   The record is MOVED to the lost table and the active slot returns to FREE,
%   so a LOST record cannot participate in association - Track_Association
%   iterates the active table only and therefore needed no change.
%
% LOST retention (frozen, literal)
%   delete when TimeSinceUpdate >= T_LOST = 1.5 s.
%   NOTE: TimeSinceUpdate accumulates from the track's LAST UPDATE, not from
%   the moment it became LOST, so this gives 1.5 s of total post-update
%   retention rather than 1.5 s in addition to the coasting phase. This is the
%   literal frozen rule; the measured consequence is reported at the checkpoint.
%
% REACQUISITION - two different things
%   1. COASTED gets a match  -> CONFIRMED, SAME TrackID. Counted in NumReacquired.
%   2. A LOST object physically reappears -> must become a NEW track with a NEW
%      TrackID. NOT IMPLEMENTABLE HERE: recognising that a detection corresponds
%      to a lost record requires comparing it against the lost table, which is
%      association with LOST records and is explicitly forbidden. No flag is
%      fabricated. Reported as an open item.
%
% TrackID is uint32, monotonic, never reused, independent of slot index. A
% deleted or lost record never returns its ID to circulation.
%
% NO EVICTION anywhere: neither the active table nor the lost table ever removes
% an existing record to make room. Overflow is reported instead.
%
% SCENARIO INDEPENDENCE: consumes only track state, covariance and timing. No
% actor identity, class, count, trajectory, map or scenario geometry.

MAX_T  = 512;
MAX_L  = 512;          % MAX_TRACKS_LOST
NCOL_L = 10;
DT     = 0.1;
KGATE  = 3.03;
WLANE  = 3.5;
T_LOST = 1.5;
V_CONV = 0.875;

ST_FREE = uint8(0); ST_TENT = uint8(1); ST_CONF = uint8(2); ST_COAST = uint8(3);

oState  = zeros(MAX_T,4);
oCov    = zeros(MAX_T,10);
oID     = zeros(MAX_T,1,'uint32');
oStatus = zeros(MAX_T,1,'uint8');
oHits   = zeros(MAX_T,1,'uint32');
oTsu    = zeros(MAX_T,1);
oR1     = zeros(MAX_T,3);
% ---- additive: persistent LiDAR extent attributes, and the ICE-facing output --
% oAttr           [512x3]  state fed back through the Unit Delay
% oTrackAttributes[512x4]  Valid | Length | Width | TrustFlags
% A freed slot falls through the ~keep continue below, so BOTH arrays stay
% exactly zero for it. No extent is invented and no default size substituted.
oAttr            = zeros(MAX_T,3);
oTrackAttributes = zeros(MAX_T,4);
oWin    = zeros(MAX_T,1,'uint32');
oAge    = zeros(MAX_T,1,'uint32');
oLost   = zeros(MAX_L,NCOL_L);
oNextID = iNextID;
lifeDiag = zeros(1,12);

% ---- 1. age the lost table and retire expired records --------------------
nLostDel = 0;
for k = 1:MAX_L
    if prevLost(k,1) == 0
        continue                            % free lost slot
    end
    tsuL = prevLost(k,9) + DT;
    if tsuL >= T_LOST
        nLostDel = nLostDel + 1;            % retired; TrackID never returns
        continue
    end
    for c = 1:NCOL_L
        oLost(k,c) = prevLost(k,c);
    end
    oLost(k,9) = tsuL;
end

% ---- 2. lifecycle transitions on the active table ------------------------
nTent = 0; nConf = 0; nCoast = 0; nDelT = 0; nConfTr = 0; nReacq = 0;
nToLost = 0; lostOvf = 0; nLostDrop = 0; nConv = 0; nExpOnEntry = 0;

for t = 1:MAX_T
    st = iStatus(t);
    if st == ST_FREE
        continue                            % slot stays entirely zero
    end

    matched = 0;
    if iTsu(t) == 0
        matched = 1;
    end
    w  = bitand(bitshift(uint32(prevWin(t)),1) + uint32(matched), uint32(7));
    ag = prevAge(t) + uint32(1);
    pc = bitand(w,uint32(1)) + bitand(bitshift(w,-1),uint32(1)) + bitand(bitshift(w,-2),uint32(1));

    keep = true;
    toLost = false;

    if st == ST_TENT
        if pc >= 2
            st = ST_CONF; nConfTr = nConfTr + 1;
        elseif (ag >= 2 && bitand(w,uint32(3)) == 0) || (ag >= 3 && pc < 2)
            keep = false; nDelT = nDelT + 1;
        end
    elseif st == ST_CONF
        if matched == 0
            st = ST_COAST;
        end
    else                                    % ST_COAST
        if matched == 1
            st = ST_CONF; nReacq = nReacq + 1;
        end
    end

    if keep && st == ST_COAST
        s1 = iCov(t,1); s2 = iCov(t,5);
        sm = s1; if s2 > sm, sm = s2; end
        if sm < 0, sm = 0; end
        if KGATE*sqrt(sm) >= WLANE
            toLost = true; keep = false;
        end
    end

    if toLost && iTsu(t) >= T_LOST
        % already past the retention limit at the moment of transfer - the
        % literal rule retires it immediately rather than holding it a frame
        nLostDel = nLostDel + 1;
        nExpOnEntry = nExpOnEntry + 1;
        toLost = false;
    end

    if toLost
        slot = 0;
        for k = 1:MAX_L
            if oLost(k,1) == 0, slot = k; break; end
        end
        if slot == 0
            lostOvf = 1; nLostDrop = nLostDrop + 1;   % NEVER evict an existing record
        else
            oLost(slot,1)  = double(iID(t));
            oLost(slot,2)  = iState(t,1);
            oLost(slot,3)  = iState(t,2);
            oLost(slot,4)  = iState(t,3);
            oLost(slot,5)  = iState(t,4);
            oLost(slot,6)  = iCov(t,1);
            oLost(slot,7)  = iCov(t,5);
            oLost(slot,8)  = iCov(t,2);
            oLost(slot,9)  = iTsu(t);
            oLost(slot,10) = double(ag);
            nToLost = nToLost + 1;
        end
    end

    if ~keep
        continue                            % slot returns to FREE (all zeros)
    end

    for c = 1:4,  oState(t,c) = iState(t,c); end
    for c = 1:10, oCov(t,c)   = iCov(t,c);   end
    for c = 1:3,  oR1(t,c)    = iR1(t,c);    end
    for c = 1:3,  oAttr(t,c)  = iAttr(t,c);  end
    oTrackAttributes(t,1) = 1;                  % Valid == post-lifecycle validity
    oTrackAttributes(t,2) = iAttr(t,1);         % Length
    oTrackAttributes(t,3) = iAttr(t,2);         % Width
    oTrackAttributes(t,4) = iAttr(t,3);         % TrustFlags, carried verbatim
    oID(t)     = iID(t);
    oStatus(t) = st;
    oHits(t)   = iHits(t);
    oTsu(t)    = iTsu(t);
    oWin(t)    = w;
    oAge(t)    = ag;

    if st == ST_TENT,  nTent  = nTent  + 1; end
    if st == ST_CONF,  nConf  = nConf  + 1; end
    if st == ST_COAST, nCoast = nCoast + 1; end
    if sqrt(iCov(t,8)) < V_CONV && sqrt(iCov(t,10)) < V_CONV
        nConv = nConv + 1;                  % derived, never a lifecycle criterion
    end
end

nLostNow = 0;
for k = 1:MAX_L
    if oLost(k,1) ~= 0, nLostNow = nLostNow + 1; end
end

lifeDiag(1)  = nTent;
lifeDiag(2)  = nConf;
lifeDiag(3)  = nCoast;
lifeDiag(4)  = nLostNow;
lifeDiag(5)  = nDelT + nLostDel;
lifeDiag(6)  = nDelT;
lifeDiag(7)  = nConfTr;
lifeDiag(8)  = nReacq;
lifeDiag(9)  = nToLost;
lifeDiag(10) = lostOvf;
lifeDiag(11) = nLostDrop;
lifeDiag(12) = nConv;

end

== matlab function ADAS_Main_ClosedLoop/Tracking_Prediction/Track_History ==
  data: trkState input; hist output; trkID input; trkStatus input; trkTsu input; simTime input; prevHist input double size=512 30 4; prevRing input uint32 size=512 1; ringIdx output; validCount output; histSpan output
function [hist, ringIdx, validCount, histSpan] = ...
    Track_History(trkState, trkID, trkStatus, trkTsu, simTime, prevHist, prevRing)
%#codegen
% TRACK_HISTORY  Stage 6: per-track temporal history ONLY.
%
% THIS BLOCK DOES NOT: estimate acceleration, emit prediction horizons, run
% Behavior/Intention, Risk, Planning or Controller, observe velocity, or do any
% LOST-track re-identification. It does not touch the state estimate, the
% lifecycle, or any Stage-3/4/5 contract - it only records where each active
% track has been.
%
% Tracking's own recursive estimator needs no history. This buffer exists to
% give Behavior/Intention temporal information downstream.
%
% LAYOUT (frozen)
%   hist [512 x 30 x 4] double   channel 1 = X
%                                channel 2 = Y
%                                channel 3 = Valid (1 measured, 0 predicted)
%                                channel 4 = timestamp (s, actual sim time)
%   30 samples at dt = 0.1 s  ->  3.0 s of coverage.
%   ringIdx [512 x 1] uint32     index of the MOST RECENT sample, 1..30; 0 = empty
%
% RING BEHAVIOUR
%   The ring advances EVERY frame for every active track, whether or not a
%   measurement arrived. The temporal grid therefore stays uniform:
%   t, t-dt, t-2dt, ... Valid samples are never compacted together, so a gap
%   remains visible as a run of Valid = 0 rather than being closed up.
%   On the 31st write the oldest sample is overwritten deterministically.
%
% VALID
%   Valid = 1 only when the track received a measurement this frame, detected as
%   trkTsu == 0 (Track_Update zeroes it on a successful update and on birth).
%   A COASTED track - or a TENTATIVE track that missed - still gets a sample
%   written with its PREDICTED X/Y, but marked Valid = 0. A prediction is never
%   recorded as a measurement.
%
% STATUS INDEPENDENCE
%   Storage does not depend on confirmation status. TENTATIVE, CONFIRMED and
%   COASTED tracks all keep history. History is never deleted for being
%   unconfirmed, and never ranked or filtered - every active slot has its own
%   independent buffer.
%
% FREE SLOTS AND SLOT REUSE
%   A slot whose status is FREE has its entire history zeroed and ringIdx set to
%   0. Because Track_Lifecycle frees a slot in the very output this block
%   consumes, the FREE state is always observed before any new track can occupy
%   that slot, so a new occupant always starts from a cleared buffer. Old and
%   new trajectories are therefore never spliced.
%
% LOST
%   A track entering LOST leaves the active table, so its slot reads FREE here
%   and its history is discarded. No history is kept for LOST records and none
%   is ever carried into a future track.
%
% TrackID vs SLOT
%   History follows the SLOT. trkID is carried only so downstream can label the
%   buffer; it is never assumed equal to the slot index.
%
% DERIVED METADATA (the only two exposed at this stage)
%   validCount [512 x 1]  number of Valid == 1 samples, 0..30. Coasted and
%                         empty samples are NOT counted.
%   histSpan   [512 x 1]  newest valid timestamp minus oldest valid timestamp,
%                         computed from the STORED TIMESTAMPS, not from the
%                         valid-sample count. Fewer than two valid samples -> 0.
%                         So valid,valid,invalid,invalid,valid spans 0.4 s, not
%                         the 0.2 s a count-based formula would give.
%
% SCENARIO INDEPENDENCE: consumes only track state, status, timing and the
% simulation clock. No actor identity, class, count, map or scenario geometry.

MAX_T = 512;
NS    = 30;

hist       = zeros(MAX_T, NS, 4);
ringIdx    = zeros(MAX_T, 1, 'uint32');
validCount = zeros(MAX_T, 1);
histSpan   = zeros(MAX_T, 1);

ts = simTime;
if ~isfinite(ts), ts = 0; end

for t = 1:MAX_T
    if trkStatus(t) == 0
        continue                    % FREE: history and ring stay exactly zero
    end

    % ---- advance the ring every frame, measured or not
    ri = double(prevRing(t)) + 1;
    if ri > NS, ri = 1; end
    if ri < 1,  ri = 1; end

    for s = 1:NS
        for c = 1:4
            hist(t,s,c) = prevHist(t,s,c);
        end
    end

    vflag = 0;
    if trkTsu(t) == 0
        vflag = 1;                  % measured this frame
    end
    hist(t,ri,1) = trkState(t,1);
    hist(t,ri,2) = trkState(t,2);
    hist(t,ri,3) = vflag;
    hist(t,ri,4) = ts;
    ringIdx(t)   = uint32(ri);

    % ---- derived metadata, from the stored timestamps
    nv = 0; tmin = 0; tmax = 0; first = true;
    for s = 1:NS
        if hist(t,s,3) == 1
            nv = nv + 1;
            tv = hist(t,s,4);
            if first
                tmin = tv; tmax = tv; first = false;
            else
                if tv < tmin, tmin = tv; end
                if tv > tmax, tmax = tv; end
            end
        end
    end
    validCount(t) = nv;
    if nv >= 2
        histSpan(t) = tmax - tmin;
    else
        histSpan(t) = 0;
    end
end

end
